simulink library "DC_Motor"  (R2017b)
settings: Solver=VariableStepAuto  StartTime=0.0  StopTime=10.0  RelTol=1e-3
values from neighbouring files (symbols this model uses):
  b = 0.002953    [PID_DC_Motor.m]    (also in data.m = rand(1,1000); data.mat = [0.0316893001122 0.642339157083 0.566870912761 0.37640954545; matlab.m = [0.031689300112206942 0.64233915708296452 0.5668709127606456)
  J = 0.02215    [PID_DC_Motor.m]
  K = 1.976    [PID_DC_Motor.m]
  L = 0.1215    [PID_DC_Motor.m]
  R = 11.2    [PID_DC_Motor.m]
settings Model: Creator=AMAN  LastModifiedBy=AMAN

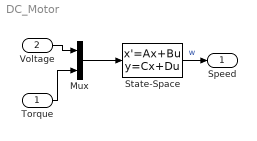
== system DC_Motor ==
  Torque : Inport
  Voltage : Inport  Port=2
  Mux : Mux  Inputs=2
  State-Space : StateSpace  A=[-b/J K/J; -K/L -R/L]  B=[0 -1/J; 1/L 0]  C=[1 0]  D=[0 0]  InitialCondition=0
  Speed : Outport
  wires:
  Mux/1 -> State-Space/1
  Voltage/1 -> Mux/1
  Torque/1 -> Mux/2
  State-Space/1 -> Speed/1  "w"
